simulink library "libAircraftMoISpecs"  (R2020b)
settings: Solver=VariableStepAuto  StartTime=0.0  StopTime=10.0  RelTol=1e-3
undefined symbols (not defined in the file): data
settings Model: Creator=caatay  LastModifiedBy=caatay

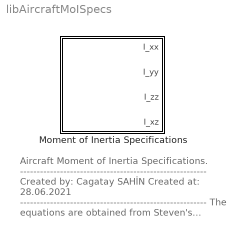
== system libAircraftMoISpecs ==
  note: Aircraft Moment of Inertia
      | Specifications.
      | --------------------------------------------------------
      | Created by: Cagatay SAHİN
      | Created at: 28.06.2021
      | --------------------------------------------------------
      | The equations are obtained from
      | Steven's textbook.
      | The reference book can be found in
      | "references folder".
      | --------------------------------------------------------
      | for question:
      | cagataysahin44@gmail.com
  Moment of Inertia Specifications : Subsystem  mask(Aircraft Specifications - Inertia Specifications){I_xx=data.acSpec.inertia.I_xx, I_yy=data.acSpec.inertia.I_yy, I_zz=data.acSpec.inertia.I_zz, I_xz=data.acSpec.inertia.I_xz}
      mask prompts: I_xx "Moment of Inertia on X-Axis"; I_yy "Moment of Inertia on Y-Axis"; I_zz "Moment of Inertia on Z-Axis"; I_xz "Moment of Inertia on XZ-Plane"
      mask help: Aircraft's moment of inertia specifications around x-y-z axis and x-z plane in Imperic format.
      mask Help:
      | This block is used for getting moment of inertia at x,y,z axis and xz plane.
      | --------------------------------------------------------------------------------------------------------------------------------------------------
      | Output of the function:
      | 	I_ii: Moment of Inertias at around axis and planes
      | --------------------------------------------------------------------------------------------------------------------------------------------------
      | All equations can be found in Steven's text book. Reference can be found in "literature" subfolder.
      | for question: "cagataysahin44@gmail.com"
      mask Display:
      | port_label('output',1,'I_{xx}','texmode','on');
      | port_label('output',2,'I_{yy}','texmode','on');
      | port_label('output',3,'I_{zz}','texmode','on');
      | port_label('output',4,'I_{xz}','texmode','on');

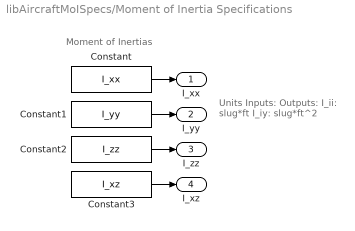
== system libAircraftMoISpecs/Moment of Inertia Specifications ==
  note: Moment of Inertias
  note: Units
      | Inputs:
      |
      | Outputs:
      | I_ii: slug*ft
      | I_iy: slug*ft^2
  Constant : Constant  Value=I_xx
  Constant1 : Constant  Value=I_yy
  Constant2 : Constant  Value=I_zz
  Constant3 : Constant  Value=I_xz
  I_xx : Outport  VectorParamsAs1DForOutWhenUnconnected=off
  I_yy : Outport  Port=2  VectorParamsAs1DForOutWhenUnconnected=off
  I_zz : Outport  Port=3  VectorParamsAs1DForOutWhenUnconnected=off
  I_xz : Outport  Port=4  VectorParamsAs1DForOutWhenUnconnected=off
  wires:
  Constant1/1 -> I_yy/1
  Constant3/1 -> I_xz/1
  Constant/1 -> I_xx/1
  Constant2/1 -> I_zz/1
